simulink model "sim1"  (R2014b)
settings: Solver=ode15s  StartTime=0.0  StopTime=10.0  MaxStep=0.01  RelTol=1e-3
undefined symbols (not defined in the file or in its folder): sigbuilder_block
settings Model: Creator=Daniel  LastModifiedBy=danielpihlquist

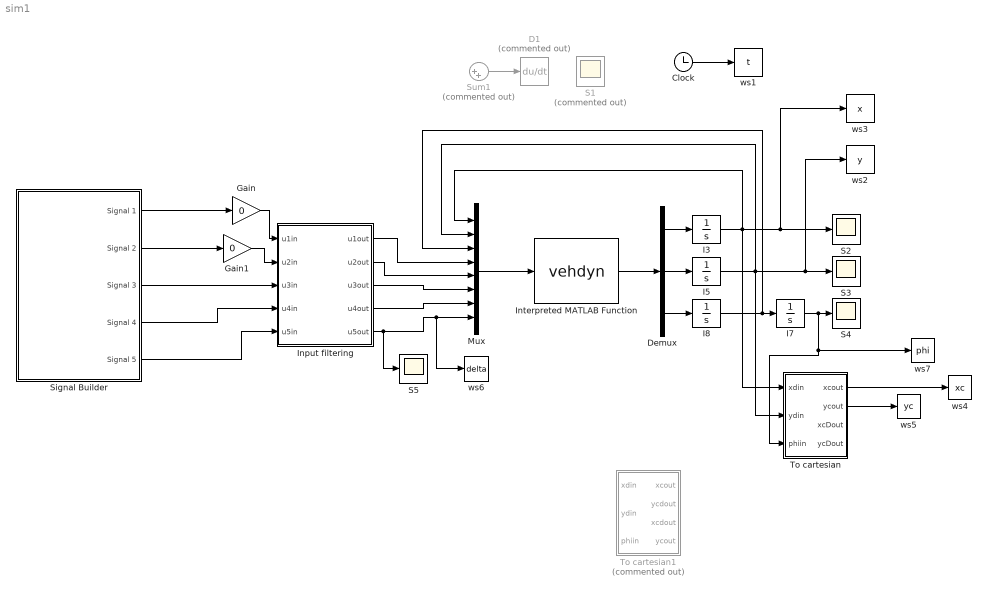
== system sim1 ==
  Clock : Clock
  D1 : Derivative  Commented=on
  Demux : Demux  Outputs=3
  Gain : Gain  Gain=0
  Gain1 : Gain  Gain=0
  I3 : Integrator  InitialCondition=10
  I5 : Integrator
  I7 : Integrator
  I8 : Integrator
  Input filtering : Subsystem
  Interpreted MATLAB Function : MATLABFcn  MATLABFcn=vehdyn
  Mux : Mux  Inputs=8
  S1 : Scope  Commented=on
  S{2..5} (4 alike) : Scope
      S2 settings: YMin=1  YMax=1.00002
      S3 settings: YMin=1  YMax=3.5  SaveName=ScopeData2
      S4 settings: YMin=-4e-06  YMax=1e-06  SaveName=ScopeData3
      S5 settings: YMin=1  YMax=1.00002  SaveName=ScopeData4
  Signal Builder : Subsystem  Tag=STV Subsys  LoadFcn=sigbuilder_block('load');  StartFcn=sigbuilder_block('start');  StopFcn=sigbuilder_block('stop');  ClipboardFcn=sigbuilder_block('clipboard');  mask(Sigbuilder block){}
      mask help: Simulink:masks:SigbuilderBlock_MD
      mask init:
      | if ~strcmp(get_param(bdroot(gcbh),'SimulationStatus'),'stopped') tuvar = sigbuilder_block('maskInit'); end
      settings: CopyFcn=sigbuilder_block('copy');  DeleteFcn=sigbuilder_block('delete');  ModelCloseFcn=sigbuilder_block('modelClose');  PreSaveFcn=sigbuilder_block('preSave');  PauseFcn=sigbuilder_block('pause');  ContinueFcn=sigbuilder_block('continue');  NameChangeFcn=sigbuilder_block('namechange');  OpenFcn=sigbuilder_block('open',[437.6 199.2 550.4 400 ]);  CloseFcn=sigbuilder_block('close');
      mask Display: plot(0, 0, 100, 100,[2, 2, 32, 32, 2], [68, 8, 8, 68, 68],[32, 2], [38, 38], [32, 19, 2],[53, 60, 44], [32, 17, 17, 2],[16, 16, 31, 31]);txt = getActiveGroup(gcbh);text(2, 100, txt,'verticalAlignment', 'top');
  Sum1 : Sum  Commented=on  Inputs=|++
  To cartesian : Subsystem
  To cartesian1 : Subsystem  Commented=on
  ws1 : ToWorkspace  VariableName=t  SampleTime=-1
  ws2 : ToWorkspace  VariableName=y  SampleTime=-1
  ws3 : ToWorkspace  VariableName=x  SampleTime=-1
  ws4 : ToWorkspace  VariableName=xc  SampleTime=-1
  ws5 : ToWorkspace  VariableName=yc  SampleTime=-1
  ws6 : ToWorkspace  VariableName=delta  SampleTime=-1
  ws7 : ToWorkspace  VariableName=phi  SampleTime=-1
  wires:
  Clock/1 -> ws1/1
  Interpreted MATLAB Function/1 -> Demux/1
  I3/1 -> S2/1, ws3/1, To cartesian/1(xdin), Mux/1
  Demux/2 -> I5/1
  Demux/1 -> I3/1
  I5/1 -> S3/1, ws2/1, To cartesian/2(ydin), Mux/2
  I8/1 -> Mux/3, I7/1
  Demux/3 -> I8/1
  I7/1 -> ws7/1, To cartesian/3(phiin), S4/1
  Sum1/1 -> D1/1
  Mux/1 -> Interpreted MATLAB Function/1
  Input filtering/1(u1out) -> Mux/4
  Input filtering/2(u2out) -> Mux/5
  Input filtering/3(u3out) -> Mux/6
  Input filtering/4(u4out) -> Mux/7
  Signal Builder/3(Signal 3) -> Input filtering/3(u3in)
  Signal Builder/4(Signal 4) -> Input filtering/4(u4in)
  Signal Builder/5(Signal 5) -> Input filtering/5(u5in)
  To cartesian/1(xcout) -> ws4/1
  To cartesian/2(ycout) -> ws5/1
  Input filtering/5(u5out) -> S5/1, ws6/1, Mux/8
  Signal Builder/2(Signal 2) -> Gain1/1
  Gain1/1 -> Input filtering/2(u2in)
  Gain/1 -> Input filtering/1(u1in)
  Signal Builder/1(Signal 1) -> Gain/1

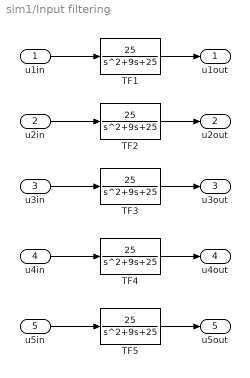
== system sim1/Input filtering ==
  u1in : Inport
  u2in : Inport  Port=2
  u3in : Inport  Port=3
  u4in : Inport  Port=4
  u5in : Inport  Port=5
  TF{1..5} (5 alike) : TransferFcn  Numerator=[25]  Denominator="[1  9 25]"
  u1out : Outport
  u2out : Outport  Port=2
  u3out : Outport  Port=3
  u4out : Outport  Port=4
  u5out : Outport  Port=5
  wires:
  TF2/1 -> u2out/1
  u1in/1 -> TF1/1
  u2in/1 -> TF2/1
  TF1/1 -> u1out/1
  TF5/1 -> u5out/1
  TF4/1 -> u4out/1
  TF3/1 -> u3out/1
  u3in/1 -> TF3/1
  u4in/1 -> TF4/1
  u5in/1 -> TF5/1

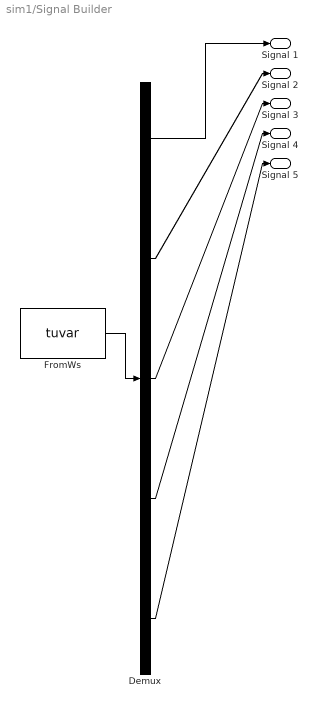
== system sim1/Signal Builder ==
  Demux : Demux  Tag=STV Demux  Outputs=5
  FromWs : FromWorkspace  Tag=STV FromWs  VariableName=tuvar  SampleTime=0
      SigBuilderData=|
      | common.afterFinalStr = 'Extrapolate'
      | common.sampleTime = 0
      | dataSet.timeRange = [0 10]
      | dataSet.name = 'Group 1'
      | sbobj.Groups.Name = 'Group 1'
      | sbobj.Groups.Signals(1).Name = 'Signal 1'
      | sbobj.Groups.Signals(1).XData = [0 1 1 2 2 10]
      | sbobj.Groups.Signals(1).YData = [0 0 1 1 0 0]
      | sbobj.Groups.Signals(2).Name = 'Signal 2'
      | sbobj.Groups.Signals(2).XData = [0 1 1 2 2 10]
      | sbobj.Groups.Signals(2).YData = [0 0 1 1 0 0]
      | sbobj.Groups.Signals(3).Name = 'Signal 3'
      | sbobj.Groups.Signals(3).XData = [0 5 6 10]
      | sbobj.Groups.Signals(3).YData = [0 0 0 0]
      | sbobj.Groups.Signals(4).Name = 'Signal 4'
      | sbobj.Groups.Signals(4).XData = [0 5 6 10]
      | sbobj.Groups.Signals(4).YData = [0 0 0 0]
      | sbobj.Groups.Signals(5).Name = 'Signal 5'
      | sbobj.Groups.Signals(5).XData = [0 2.52 2.52 4.42 4.42 5 5.83333333333 6.66666666667 7.5 7.5 8.33333333333 8.33333333333 9.16666666667 10]
      | sbobj.Groups.Signals(5).YData = [0 0 0.1 0.1 0 0 0 0 0 -0.1 -0.1 0 0 0]
  Signal 1 : Outport  Tag=STV Outport
  Signal 2 : Outport  Tag=STV Outport  Port=2
  Signal 3 : Outport  Tag=STV Outport  Port=3
  Signal 4 : Outport  Tag=STV Outport  Port=4
  Signal 5 : Outport  Tag=STV Outport  Port=5
  wires:
  Demux/1 -> Signal 1/1
  FromWs/1 -> Demux/1
  Demux/2 -> Signal 2/1
  Demux/3 -> Signal 3/1
  Demux/4 -> Signal 4/1
  Demux/5 -> Signal 5/1

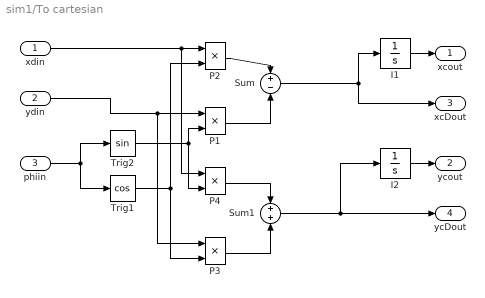
== system sim1/To cartesian ==
  xdin : Inport
  ydin : Inport  Port=2
  phiin : Inport  Port=3
  I1 : Integrator  InitialCondition=1
  I2 : Integrator  InitialCondition=1
  P{1..4} (4 alike) : Product
  Sum : Sum  Inputs=+|-
  Sum1 : Sum  Inputs=+|+
  Trig1 : Trigonometry  Operator=cos
  Trig2 : Trigonometry
  xcout : Outport
  ycout : Outport  Port=2
  xcDout : Outport  Port=3
  ycDout : Outport  Port=4
  wires:
  phiin/1 -> Trig2/1, Trig1/1
  I2/1 -> ycout/1
  I1/1 -> xcout/1
  P2/1 -> Sum/1
  P1/1 -> Sum/2
  P4/1 -> Sum1/1
  P3/1 -> Sum1/2
  Trig1/1 -> P2/2, P3/2
  xdin/1 -> P4/1, P2/1
  Trig2/1 -> P4/2, P1/2
  ydin/1 -> P3/1, P1/1
  Sum1/1 -> I2/1, ycDout/1
  Sum/1 -> xcDout/1, I1/1

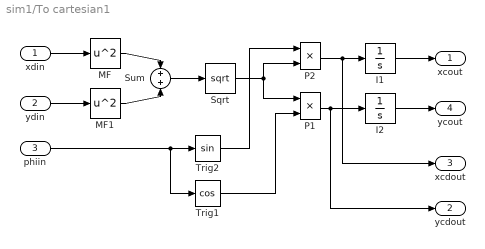
== system sim1/To cartesian1 ==
  xdin : Inport
  ydin : Inport  Port=2
  phiin : Inport  Port=3
  I1 : Integrator  InitialCondition=1
  I2 : Integrator  InitialCondition=1
  MF : Math  Operator=square  SaturateOnIntegerOverflow=on
  MF1 : Math  Operator=square  SaturateOnIntegerOverflow=on
  P1 : Product
  P2 : Product
  Sqrt : Sqrt  SaturateOnIntegerOverflow=on
  Sum : Sum  Inputs=+|+
  Trig1 : Trigonometry  Operator=cos
  Trig2 : Trigonometry
  xcout : Outport
  ycdout : Outport  Port=2
  xcdout : Outport  Port=3
  ycout : Outport  Port=4
  wires:
  I1/1 -> xcout/1
  I2/1 -> ycout/1
  P2/1 -> I1/1, xcdout/1
  P1/1 -> I2/1, ycdout/1
  Trig1/1 -> P1/2
  Trig2/1 -> P2/1
  Sqrt/1 -> P2/2, P1/1
  phiin/1 -> Trig2/1, Trig1/1
  Sum/1 -> Sqrt/1
  MF1/1 -> Sum/2
  MF/1 -> Sum/1
  ydin/1 -> MF1/1
  xdin/1 -> MF/1
